simulink model "pendulum"  (R2023b)
settings: Solver=VariableStepAuto  StartTime=0.0  StopTime=10.0  MaxStep=1e-3  RelTol=1e-3
undefined symbols (not defined in the file): I
libraries: simulink_extras x2
settings Model: Creator=B03-304  LastModifiedBy=B03-304

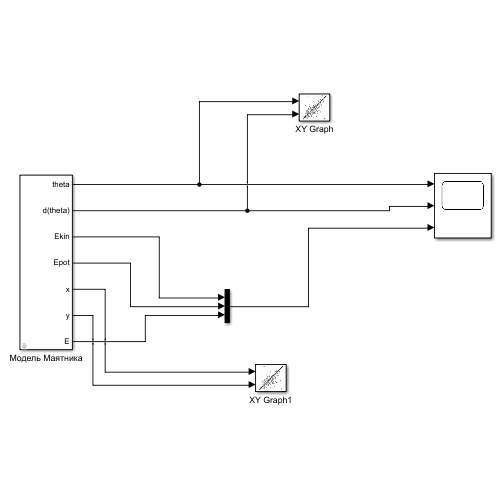
[thumbnail: Simulink's stored preview of the top-level diagram]
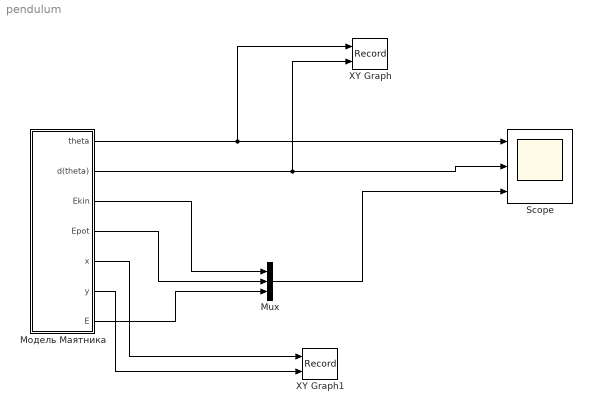
== system pendulum ==
  Mux : Mux  Inputs=3
  Scope : Scope  NumInputPorts=3
  XY Graph : Record  FileSettingsInternal="{\"entries\":[{\"content\":{\"excelSettings\":{\"content\":{},\"type\":\"Streamout.ExcelSettings\"}},\"type\":\"Streamout.FileSettingStorage\",\"uuid\":\"\"}],\"packageUris\":[\"http:\\/\\/schema.mathworks.com\\/mf0\\/streamout_blocks\\/R2020a\"],\"version\":\"1.0\"}"  Layout=[1 1]  SignalsInternal="{\"entries\":[{\"content\":{\"signals\":[{\"content\":{\"blockPath\":[],\"dimensions\":[1],\"domain\":\"\",\"lineColor\":\"#a2142f\",\"plots\":[1],\"port\":1,\"sid\":[\"\"],\"signalID\":120,\"signalName\":\"Модель Маятника:1\"},\"type\":\"RecordBlkView.Signal\",\"uuid\":\"\"},{\"content\":{\"blockPath\":[],\"dimensions\":[1],\"domain\":\"\",\"lineColor\":\"#139fff\",\"plots\":[1],\"port\":2,\"sid\":[\"\"],\"signalID\":124,\"signalName\":\"Модель Маятника:2\"},\"type\":\"RecordBlkView.Signal\",\"uuid\":\"\"}]},\"type\":\"RecordBlkView.InputSignals\",\"uuid\":\"\"}],\"packageUris\":[\"http:\\/\\/schema.mathworks.com\\/mf0\\/streamout_blocks\\/R2020a\"],\"version\":\"1.0\"}"  VisualizationBindings="{\"xyplotplugin\":{\"info\":[{\"series\":[{\"bindingParametersList\":[{\"parameter\":\"X-Axis\",\"signalID\":120,\"signalName\":\"Модель Маятника:1\"},{\"parameter\":\"Y-Axis\",\"signalID\":124,\"signalName\":\"Модель Маятника:2\"}],\"seriesID\":57637}],\"subplotID\":1}]}}"  CompatibilityTag=XY
  XY Graph1 : Record  FileSettingsInternal="{\"entries\":[{\"content\":{\"excelSettings\":{\"content\":{},\"type\":\"Streamout.ExcelSettings\"}},\"type\":\"Streamout.FileSettingStorage\",\"uuid\":\"\"}],\"packageUris\":[\"http:\\/\\/schema.mathworks.com\\/mf0\\/streamout_blocks\\/R2020a\"],\"version\":\"1.0\"}"  Layout=[1 1]  SignalsInternal="{\"entries\":[{\"content\":{\"signals\":[{\"content\":{\"blockPath\":[],\"dimensions\":[1],\"domain\":\"\",\"lineColor\":\"#a2142f\",\"plots\":[1],\"port\":1,\"sid\":[\"\"],\"signalID\":128,\"signalName\":\"Модель Маятника:5\"},\"type\":\"RecordBlkView.Signal\",\"uuid\":\"\"},{\"content\":{\"blockPath\":[],\"dimensions\":[1],\"domain\":\"\",\"lineColor\":\"#139fff\",\"plots\":[1],\"port\":2,\"sid\":[\"\"],\"signalID\":132,\"signalName\":\"Модель Маятника:6\"},\"type\":\"RecordBlkView.Signal\",\"uuid\":\"\"}]},\"type\":\"RecordBlkView.InputSignals\",\"uuid\":\"\"}],\"packageUris\":[\"http:\\/\\/schema.mathworks.com\\/mf0\\/streamout_blocks\\/R2020a\"],\"version\":\"1.0\"}"  VisualizationBindings="{\"xyplotplugin\":{\"info\":[{\"series\":[{\"bindingParametersList\":[{\"parameter\":\"X-Axis\",\"signalID\":128,\"signalName\":\"Модель Маятника:5\"},{\"parameter\":\"Y-Axis\",\"signalID\":132,\"signalName\":\"Модель Маятника:6\"}],\"seriesID\":41878}],\"subplotID\":1}]}}"  CompatibilityTag=XY
  Модель Маятника : Subsystem  mask{thtea0=pi/6, b=0, m=2, l=1, g=9.8}
  wires:
  Модель Маятника/1(theta) -> XY Graph/1, Scope/1
  Модель Маятника/2(d(theta)) -> XY Graph/2, Scope/2
  Mux/1 -> Scope/3
  Модель Маятника/3(Ekin) -> Mux/1
  Модель Маятника/4(Epot) -> Mux/2
  Модель Маятника/7(E) -> Mux/3
  Модель Маятника/5(x) -> XY Graph1/1
  Модель Маятника/6(y) -> XY Graph1/2

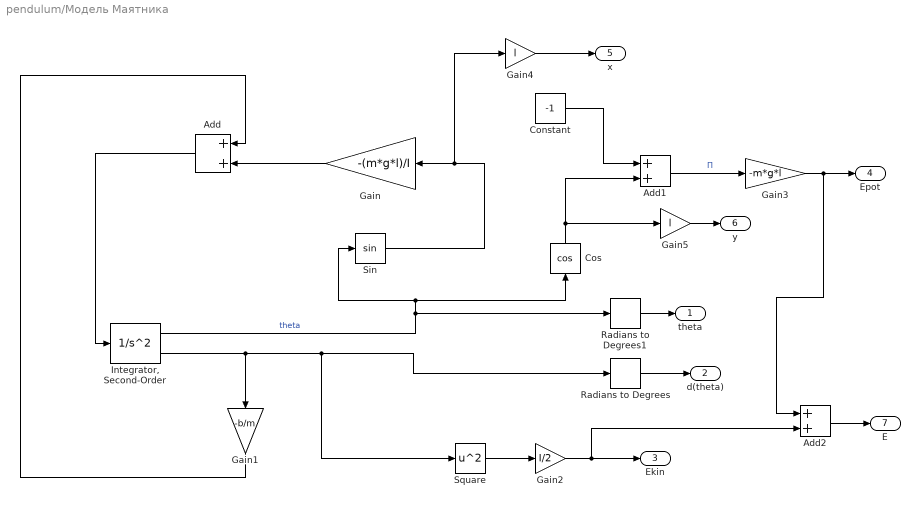
== system pendulum/Модель Маятника ==
  Add : Sum
  Add1 : Sum
  Add2 : Sum
  Constant : Constant  Value=-1
  Cos : Trigonometry  Operator=cos
  Gain : Gain  Gain=-(m*g*l)/I
  Gain1 : Gain  Gain=-b/m
  Gain2 : Gain  Gain=I/2
  Gain3 : Gain  Gain=-m*g*l
  Gain4 : Gain  Gain=l
  Gain5 : Gain  Gain=l
  "Integrator, Second-Order" : SecondOrderIntegrator  ICX=thtea0
  Radians to Degrees : simulink_extras/Transformations/Radians to Degrees
  Radians to Degrees1 : simulink_extras/Transformations/Radians to Degrees
  Sin : Trigonometry
  Square : Math  Operator=square
  theta : Outport
  d(theta) : Outport  Port=2
  Ekin : Outport  Port=3
  Epot : Outport  Port=4
  x : Outport  Port=5
  y : Outport  Port=6
  E : Outport  Port=7
  wires:
  "Integrator, Second-Order"/1 -> Cos/1, Sin/1, Radians to Degrees1/1  "theta"
  Radians to Degrees1/1 -> theta/1
  Radians to Degrees/1 -> d(theta)/1
  "Integrator, Second-Order"/2 -> Square/1, Radians to Degrees/1, Gain1/1
  Sin/1 -> Gain4/1, Gain/1
  Add/1 -> "Integrator, Second-Order"/1
  Gain/1 -> Add/2
  Gain1/1 -> Add/1
  Square/1 -> Gain2/1
  Gain2/1 -> Add2/2, Ekin/1
  Cos/1 -> Gain5/1, Add1/2
  Constant/1 -> Add1/1
  Add1/1 -> Gain3/1  "П"
  Gain3/1 -> Add2/1, Epot/1
  Gain4/1 -> x/1
  Gain5/1 -> y/1
  Add2/1 -> E/1
